simulink model "Filter_HDL_1"  (R2016a)
settings: Solver=VariableStepAuto  StartTime=0.0  StopTime=10.0  RelTol=1e-3
libraries: xbsIndex_r4 x39
settings Model: Creator=Stella Modyanto  LastModifiedBy=Stella Modyanto

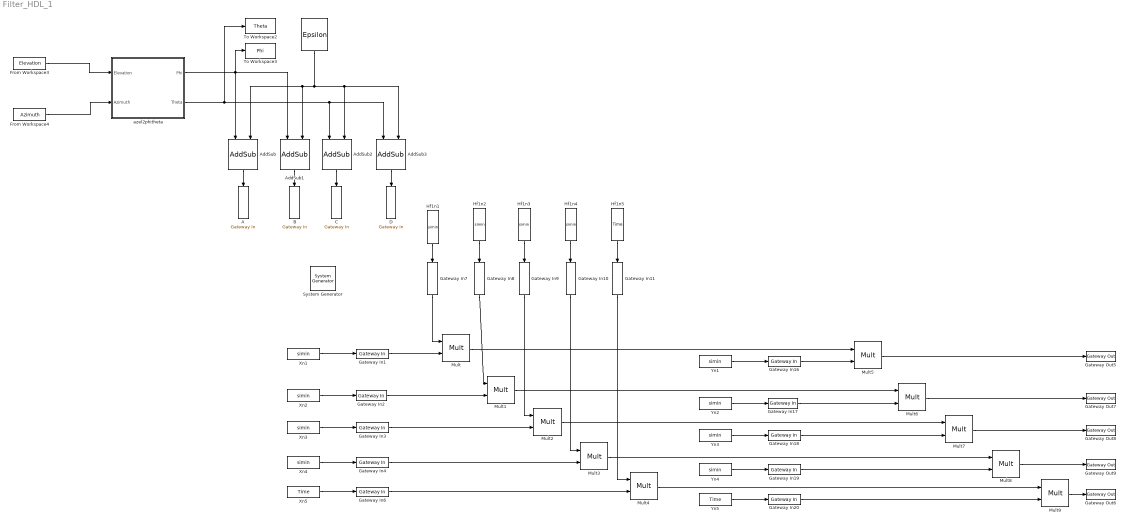
== system Filter_HDL_1 ==
  " " : FromWorkspace  VariableName=Epsilon  SampleTime=0
  " System Generator" : xbsIndex_r4/ System Generator  Tag=genX  xilinxfamily=virtex7  part=xc7vx485t  speed=-2  package=ffg1761  synthesis_tool=Vivado  clock_wrapper=Clock Enables  directory=./netlist  proj_type=Vivado  Synth_file=Vivado Synthesis Defaults  Impl_file=Vivado Implementation Defaults  testbench=off  simulink_period=1  sysclk_period=10  dcm_input_clock_period=10  incr_netlist=off  trim_vbits=Everywhere in SubSystem  dbl_ovrd=According to Block Masks  core_generation=According to Block Masks  run_coregen=off  deprecated_control=off  eval_field=0  block_type=sysgen
  A : xbsIndex_r4/Gateway In  gui_display_data_type=Fixed-point  arith_type="Signed  (2's comp)"  n_bits=16  bin_pt=14  preci_type=Single  exp_width=8  frac_width=24  rows=1  columns=1  quantization="Round  (unbiased: +/- Inf)"  overflow=Saturate  period=1  UseAsADC=off  ADCChannel='1'  interface=None  automatic_assignment=on  address_offset=hex2dec('00')  intf_name=''  intf_description=''  default_value=0  timing_constraint=None  locs_specified=off  LOCs={}  io_standard={}  inherit_from_input=off  hdl_port=on  dbl_ovrd=off  block_type=gatewayin
  AddSub : xbsIndex_r4/AddSub  mode=Addition  use_carryin=off  use_carryout=off  en=off  latency=1  precision=Full  arith_type=Unsigned  n_bits=16  bin_pt=14  quantization=Truncate  overflow=Wrap  use_behavioral_HDL=off  hw_selection=Fabric  pipelined=off  dbl_ovrd=off  block_type=addsub
  AddSub1 : xbsIndex_r4/AddSub  mode=Subtraction  use_carryin=off  use_carryout=off  en=off  latency=1  precision=Full  arith_type=Unsigned  n_bits=16  bin_pt=14  quantization=Truncate  overflow=Wrap  use_behavioral_HDL=off  hw_selection=Fabric  pipelined=off  dbl_ovrd=off  block_type=addsub
  AddSub2 : xbsIndex_r4/AddSub  mode=Addition  use_carryin=off  use_carryout=off  en=off  latency=1  precision=Full  arith_type=Unsigned  n_bits=16  bin_pt=14  quantization=Truncate  overflow=Wrap  use_behavioral_HDL=off  hw_selection=Fabric  pipelined=off  dbl_ovrd=off  block_type=addsub
  AddSub3 : xbsIndex_r4/AddSub  mode=Subtraction  use_carryin=off  use_carryout=off  en=off  latency=1  precision=Full  arith_type=Unsigned  n_bits=16  bin_pt=14  quantization=Truncate  overflow=Wrap  use_behavioral_HDL=off  hw_selection=Fabric  pipelined=off  dbl_ovrd=off  block_type=addsub
  B : xbsIndex_r4/Gateway In  gui_display_data_type=Fixed-point  arith_type="Signed  (2's comp)"  n_bits=16  bin_pt=14  preci_type=Single  exp_width=8  frac_width=24  rows=1  columns=1  quantization="Round  (unbiased: +/- Inf)"  overflow=Saturate  period=1  UseAsADC=off  ADCChannel='1'  interface=None  automatic_assignment=on  address_offset=hex2dec('00')  intf_name=''  intf_description=''  default_value=0  timing_constraint=None  locs_specified=off  LOCs={}  io_standard={}  inherit_from_input=off  hdl_port=on  dbl_ovrd=off  block_type=gatewayin
  C : xbsIndex_r4/Gateway In  gui_display_data_type=Fixed-point  arith_type="Signed  (2's comp)"  n_bits=16  bin_pt=14  preci_type=Single  exp_width=8  frac_width=24  rows=1  columns=1  quantization="Round  (unbiased: +/- Inf)"  overflow=Saturate  period=1  UseAsADC=off  ADCChannel='1'  interface=None  automatic_assignment=on  address_offset=hex2dec('00')  intf_name=''  intf_description=''  default_value=0  timing_constraint=None  locs_specified=off  LOCs={}  io_standard={}  inherit_from_input=off  hdl_port=on  dbl_ovrd=off  block_type=gatewayin
  D : xbsIndex_r4/Gateway In  gui_display_data_type=Fixed-point  arith_type="Signed  (2's comp)"  n_bits=16  bin_pt=14  preci_type=Single  exp_width=8  frac_width=24  rows=1  columns=1  quantization="Round  (unbiased: +/- Inf)"  overflow=Saturate  period=1  UseAsADC=off  ADCChannel='1'  interface=None  automatic_assignment=on  address_offset=hex2dec('00')  intf_name=''  intf_description=''  default_value=0  timing_constraint=None  locs_specified=off  LOCs={}  io_standard={}  inherit_from_input=off  hdl_port=on  dbl_ovrd=off  block_type=gatewayin
  From Workspace3 : FromWorkspace  VariableName=Elevation  SampleTime=0
  From Workspace4 : FromWorkspace  VariableName=Azimuth  SampleTime=0
  Gateway In{1..4,6..11,16..20} (15 alike) : xbsIndex_r4/Gateway In  gui_display_data_type=Fixed-point  arith_type="Signed  (2's comp)"  n_bits=16  bin_pt=14  preci_type=Single  exp_width=8  frac_width=24  rows=1  columns=1  quantization="Round  (unbiased: +/- Inf)"  overflow=Saturate  period=1  UseAsADC=off  ADCChannel='1'  interface=None  automatic_assignment=on  address_offset=hex2dec('00')  intf_name=''  intf_description=''  default_value=0  timing_constraint=None  locs_specified=off  LOCs={}  io_standard={}  inherit_from_input=off  hdl_port=on  dbl_ovrd=off  block_type=gatewayin
  Gateway Out{5..9} (5 alike) : xbsIndex_r4/Gateway Out  inherit_from_input=off  hdl_port=on  rows=1  columns=1  UseAsDAC=off  DACChannel='1'  interface=None  automatic_assignment=on  address_offset=hex2dec('00')  intf_name=''  intf_description=''  timing_constraint=None  locs_specified=off  LOCs={}  io_standard={}  block_type=gatewayout
  Hf1n{1..4} (4 alike) : FromWorkspace  VariableName=simin  SampleTime=0
  Hf1n5 : FromWorkspace  VariableName=Time  SampleTime=0
  Mult{,1..9} (10 alike) : xbsIndex_r4/Mult  precision=Full  arith_type="Signed  (2's comp)"  n_bits=16  bin_pt=14  quantization=Truncate  overflow=Wrap  en=off  latency=3  use_behavioral_HDL=off  opt=Speed  use_embedded=on  optimum_pipeline=off  pipeline=on  dbl_ovrd=off  use_rpm=on  placement_style=Triangular  block_type=mult
  To Workspace2 : ToWorkspace  VariableName=Theta  SaveFormat=Timeseries  SampleTime=-1
  To Workspace3 : ToWorkspace  VariableName=Phi  SaveFormat=Timeseries  SampleTime=-1
  "Xn1 " : FromWorkspace  VariableName=simin  SampleTime=0
  Xn2 : FromWorkspace  VariableName=simin  SampleTime=0
  "Xn3 " : FromWorkspace  VariableName=simin  SampleTime=0
  "Xn4 " : FromWorkspace  VariableName=simin  SampleTime=0
  Xn5 : FromWorkspace  VariableName=Time  SampleTime=0
  Yn{1..4} (4 alike) : FromWorkspace  VariableName=simin  SampleTime=0
  Yn5 : FromWorkspace  VariableName=Time  SampleTime=0
  "azel2phitheta " : Subsystem
  wires:
  " "/1 -> AddSub1/2, AddSub/2, AddSub2/2, AddSub3/2
  "azel2phitheta "/1(Phi) -> AddSub1/1, To Workspace3/1, AddSub/1
  "azel2phitheta "/2("Theta ") -> To Workspace2/1, AddSub2/1, AddSub3/1
  From Workspace3/1 -> "azel2phitheta "/1(Elevation)
  From Workspace4/1 -> "azel2phitheta "/2(Azimuth)
  AddSub3/1 -> D/1
  AddSub2/1 -> C/1
  AddSub1/1 -> B/1
  AddSub/1 -> A/1
  "Xn1 "/1 -> Gateway In1/1
  Xn2/1 -> Gateway In2/1
  "Xn3 "/1 -> Gateway In3/1
  "Xn4 "/1 -> Gateway In4/1
  Xn5/1 -> Gateway In6/1
  Hf1n1/1 -> Gateway In7/1
  Hf1n2/1 -> Gateway In8/1
  Hf1n3/1 -> Gateway In9/1
  Hf1n4/1 -> Gateway In10/1
  Hf1n5/1 -> Gateway In11/1
  Gateway In1/1 -> Mult/2
  Gateway In7/1 -> Mult/1
  Gateway In8/1 -> Mult1/1
  Gateway In2/1 -> Mult1/2
  Mult/1 -> Mult5/1
  Mult1/1 -> Mult6/1
  Gateway In3/1 -> Mult2/2
  Gateway In9/1 -> Mult2/1
  Gateway In10/1 -> Mult3/1
  Gateway In4/1 -> Mult3/2
  Gateway In6/1 -> Mult4/2
  Gateway In11/1 -> Mult4/1
  Mult2/1 -> Mult7/1
  Mult3/1 -> Mult8/1
  Mult4/1 -> Mult9/1
  Yn1/1 -> Gateway In16/1
  Yn2/1 -> Gateway In17/1
  Yn3/1 -> Gateway In18/1
  Yn4/1 -> Gateway In19/1
  Yn5/1 -> Gateway In20/1
  Gateway In16/1 -> Mult5/2
  Gateway In17/1 -> Mult6/2
  Mult5/1 -> Gateway Out5/1
  Mult6/1 -> Gateway Out7/1
  Gateway In18/1 -> Mult7/2
  Gateway In19/1 -> Mult8/2
  Gateway In20/1 -> Mult9/2
  Mult7/1 -> Gateway Out8/1
  Mult8/1 -> Gateway Out9/1
  Mult9/1 -> Gateway Out6/1

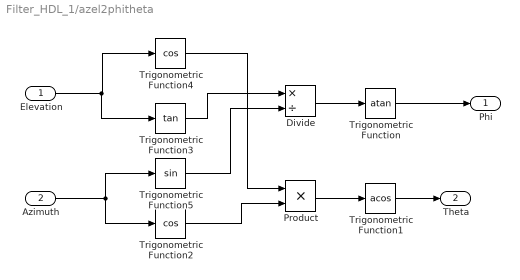
== system Filter_HDL_1/azel2phitheta  ==
  Elevation : Inport
  Azimuth : Inport  Port=2
  Divide : Product  Inputs=*/
  Product : Product
  Trigonometric Function : Trigonometry  Operator=atan
  Trigonometric Function1 : Trigonometry  Operator=acos
  Trigonometric Function2 : Trigonometry  Operator=cos
  Trigonometric Function3 : Trigonometry  Operator=tan
  Trigonometric Function4 : Trigonometry  Operator=cos
  Trigonometric Function5 : Trigonometry
  Phi : Outport
  "Theta " : Outport  Port=2
  wires:
  Azimuth/1 -> Trigonometric Function2/1, Trigonometric Function5/1
  Trigonometric Function2/1 -> Product/2
  Trigonometric Function4/1 -> Product/1
  Divide/1 -> Trigonometric Function/1
  Trigonometric Function1/1 -> "Theta "/1
  Trigonometric Function5/1 -> Divide/2
  Trigonometric Function3/1 -> Divide/1
  Product/1 -> Trigonometric Function1/1
  Elevation/1 -> Trigonometric Function3/1, Trigonometric Function4/1
  Trigonometric Function/1 -> Phi/1
